simulink model "untitled"  (R2019b)
settings: Solver=VariableStepAuto  StartTime=0.0  StopTime=1000  RelTol=1e-3
settings Model: Creator=Rashedul Islam  LastModifiedBy=Rashedul Islam

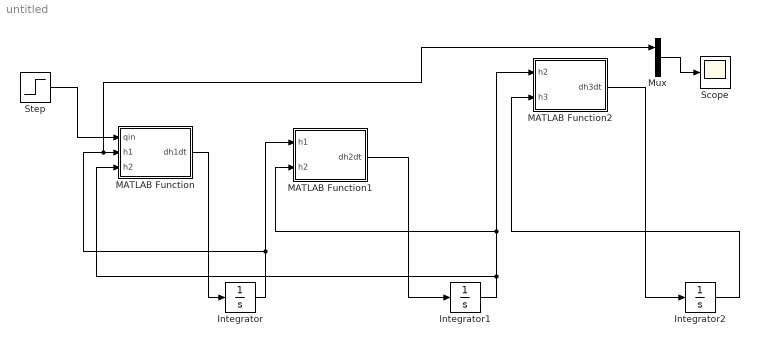
== system untitled ==
  Integrator : Integrator
  Integrator1 : Integrator
  Integrator2 : Integrator
  MATLAB Function : MATLAB Function  TreatAsAtomicUnit=on
  MATLAB Function1 : MATLAB Function  TreatAsAtomicUnit=on
  MATLAB Function2 : MATLAB Function  TreatAsAtomicUnit=on
  Mux : Mux  Inputs=3
  Scope : Scope
  Step : Step  Time=500  Before=4  After=6  SampleTime=0
  wires:
  Mux/1 -> Scope/1
  MATLAB Function2/1(dh3dt) -> Integrator2/1
  Integrator2/1 -> MATLAB Function2/2(h3)
  MATLAB Function1/1(dh2dt) -> Integrator1/1
  Integrator1/1 -> MATLAB Function/3(h2), MATLAB Function2/1(h2), MATLAB Function1/2(h2)
  MATLAB Function/1(dh1dt) -> Integrator/1
  Integrator/1 -> Mux/1, MATLAB Function/2(h1), MATLAB Function1/1(h1)
  Step/1 -> MATLAB Function/1(qin)

== matlab function untitled/MATLAB Function1 ==
  data: dh2dt output; h1 input; h2 input
function dh2dt = fcn(h1,h2)
q1= (5*abs(h1)^.5) -(5*abs(h2)^.5) ;
q2=5*abs(h2)^.5 ;
A= (pi*10^2) /4 ;

dh2dt = (q1-q2)/A;

== matlab function untitled/MATLAB Function ==
  data: qin input; dh1dt output; h1 input; h2 input
function dh1dt = fcn(qin,h1,h2)
q1= (5*abs(h1)^.5) -(5*abs(h2)^.5) ;
A= (pi*10^2) /4 ;

dh1dt = (qin-q1)/A;

== matlab function untitled/MATLAB Function2 ==
  data: h2 input; h3 input; dh3dt output
function dh3dt = fcn(h2,h3)
%q1= (5*abs(h1)^.5) -(5*abs(h2)^.5);
q2=5*abs(h2)^.5 ;
q3=5*abs(h3)^.5 ;
A= (pi*10^2) /4 ;

dh3dt = (q2-q3)/A;
